simulink model "FullModelAddANN_Final_ANN_revised"  (R2024b)
settings: Solver=ode4  StartTime=0.0  StopTime=40  FixedStep=1e-5  RelTol=1e-3
values from neighbouring files (symbols this model uses):
  Dp = 2.506338228783948e3    (= 2506.33822878)    [FullModelAddANNm_Final.m]    (also in main_opal_ann_control.m)
  Dq = 1.033099625954584    (= 1.03309962595)    [FullModelAddANNm_Final.m]    (also in main_opal_ann_control.m)
  Kp = 0.006383815167581    (= 0.00638381516758)    [FullModelAddANNm_Final.m]    (also in main_opal_ann_control.m)
  Kq = 0.076670166944346    (= 0.0766701669443)    [FullModelAddANNm_Final.m]    (also in main_opal_ann_control.m)
undefined symbols (not defined in the file or in its folder): Filter, Ls, params
libraries: neural x88, spsCurrentMeasurementLib x6, spsParallelRLCBranchLib x6, spsIGBTDiodeLib x6, spsMeanLib x6, spsSeriesRLCBranchLib x6, simulink x4, spsVoltageMeasurementLib x4, spsVariableInductorLib x3, spsVariableResistorLib x3, spsDCVoltageSourceLib x1, spsThreePhaseSourceLib x1
(part 3 of 11)

== system FullModelAddANN_Final_ANN_revised/Feed-Forward Neural Network_strength/Process Input 1 ==
  x : Inport  PortDimensions=200
      mask Display: e = 0.06;c1 = [120 230 180]/255;c2 = ([120 230 180]+0)/(256+128);c3 = ([120 230 180]+128)/(256+128);patch([0 1 1 0],[0 0 1 1],c1);patch([0 1 1 1-e 1-e 0+e],[0 0 1 1-e 0+e 0+e],c2);patch([0 0 1 1-e 0+e 0+e],[0 1 1 1-e 1-e 0+e],c3);plot([0 1 1 0 0],[0 0 1 1 0]);
  mapminmax : neural/Processing Functions/mapminmax  xmin=[-8.56223999999999918486537353601;0.341988000000000014200196574166;11.4306000000000000937916411203;18.8948999999999998067323758733;33.501600000000003376499080332;44.2207999999999969986674841493;53.7240999999999999658939486835;67.3171999999999997044142219238;78.7112999999999942701833788306;88.2877000000000009549694368616;87.0142000000000024328983272426;84.2195999999999997953636921011;75.1424999999999982946974341758;70.2459000000000060026650317013;62.8965999999999993974597600754;58.1272000000000019781509763561;53.039000000000001477928890381;47.5546000000000006480149750132;39.1567999999999969418240652885;34.2475999999999984879650583025;24.8386999999999993349319993285;21.4954000000000000625277607469;15.5536999999999991928234521765;6.39240999999999992553512129234;2.04654999999999986926013662014;-1.18479000000000000980548975349;-8.32602999999999937585926090833;-16.5778999999999996362021192908;-17.0478999999999984993337420747;-28.4237999999999999545252649114;-36.734499999999997044142219238;-41.9243999999999985561771609355;-51.339199999999998169641912682;-60.2991000000000028080648917239;-64.033100000000004570210876409;-68.9287999999999954070517560467;-74.5424000000000006593836587854;-81.1367000000000047066350816749;-86.5153999999999996362021192908;-88.4420999999999963847585604526;-95.1997000000000070940586738288;-95.5378999999999933834260446019;-99.909199999999998453859006986;-101.362999999999999545252649114;-102.371999999999999886313162278;-105.39300000000000068212102633;-108.334999999999993747223925311;-107.676000000000001932676241267;-105.603999999999999204192135949;-106.033000000000001250555214938;-109.465999999999993974597600754;-107.385000000000005115907697473;-110.787000000000006139089236967;-108.763000000000005229594535194;-111.801000000000001932676241267;-116.733999999999994656718627084;-124.862999999999999545252649114;-132.080999999999988858689903282;-139.818999999999988403942552395;-149.477000000000003865352482535;-155.419000000000011141310096718;-162.912000000000006139089236967;-172.710000000000007958078640513;-174.960000000000007958078640513;-176.641999999999995907273842022;-175.318000000000012050804798491;-171.712999999999993860910763033;-175.141999999999995907273842022;-176.205999999999988858689903282;-178.522999999999996134647517465;-178.052999999999997271515894681;-177.605999999999994543031789362;-176.187999999999988176568876952;-177.283999999999991814547684044;-176.68899999999999295141606126;-172.467999999999989313437254168;-171.126000000000004774847184308;-169.0970000000000084128259914;-171.228000000000008640199666843;-171.382000000000005002220859751;-170.621000000000009322320693173;-165.554000000000002046363078989;-158.830000000000012505552149378;-153.207999999999998408384271897;-144.509999999999990905052982271;-137.977000000000003865352482535;-128.074000000000012278178473935;-118.063000000000002387423592154;-109.509000000000000341060513165;-98.0019000000000062300387071446;-86.757999999999995566213328857;-77.2938999999999936107997200452;-68.6098999999999961119101499207;-57.2740999999999971237230056431;-49.8582999999999998408384271897;-41.8474000000000003751665644813;-34.7081999999999979422682372387;-28.5457999999999998408384271897;-22.813300000000001688249540166;-13.833600000000000562749846722;-6.93552000000000035129232855979;-5.91626000000000029643842935911;-4.71670999999999995822008713731;-4.42295000000000015916157281026;-4.29441999999999968196107147378;-3.89672000000000018360424292041;-3.41660999999999992482457855658;-2.41442999999999985405452207488;-1.00232999999999994322763541277;0.7520130000000000425330881626;2.50716999999999989867660588061;4.16727000000000025181634555338;5.89646000000000025664803615655;7.19420999999999999374722392531;7.83779000000000003467448550509;8.51986999999999916610704531195;9.02068000000000047577941586496;9.4842700000000004223466021358;9.89752000000000009549694368616;10.2754999999999991899812812335;10.6089000000000002188471626141;10.906800000000000494537744089 ...(+2559 chars)]  xmax=[111.865999999999999658939486835;112.992000000000004433786671143;112.234999999999999431565811392;109.850999999999999090505298227;113.064999999999997726263245568;118.135999999999995679900166579;124.359999999999999431565811392;132.878999999999990677679306827;140.645000000000010231815394945;148.348000000000013187673175707;156.0970000000000084128259914;164.181000000000011596057447605;170.609000000000008867573342286;175.45699999999999363353708759;177.248999999999995225152815692;173.300000000000011368683772162;172.157000000000010686562745832;173.884999999999990905052982271;176.134999999999990905052982271;177.842000000000012960299500264;176.912000000000006139089236967;178.641999999999995907273842022;178.368999999999999772626324557;179.169000000000011141310096718;175.943999999999988403942552395;173.278999999999996362021192908;172.058999999999997498889570124;169.233000000000004092726157978;171.375;170.43899999999999295141606126;171.050000000000011368683772162;164.754999999999995452526491135;159.145000000000010231815394945;152.873999999999995225152815692;144.052999999999997271515894681;135.844999999999998863131622784;127.575999999999993406163412146;118.522999999999996134647517465;110.171000000000006480149750132;98.8944999999999936335370875895;87.4979000000000013415046851151;78.2850999999999999090505298227;68.0520999999999958163243718445;57.8346999999999979991116560996;49.7299000000000006593836587854;40.7706000000000017280399333686;34.8459999999999965325514494907;29.2646000000000015006662579253;23.2098000000000013187673175707;14.4864999999999994884092302527;7.16436999999999990507149050245;-0.0668678000000000050118131866839;-8.32135000000000069064753915882;-18.791399999999999437250153278;-32.2524999999999977262632455677;-44.6839999999999974988895701244;-56.7535000000000025011104298756;-67.7192000000000007275957614183;-77.1479999999999961346475174651;-89.4813999999999936107997200452;-85.4127000000000009549694368616;-80.3586999999999989086063578725;-74.9572000000000002728484105319;-69.0717999999999960891727823764;-66.0060000000000002273736754432;-55.3436999999999983401721692644;-44.1308000000000006934897101019;-44.1448999999999998067323758733;-34.423099999999998033217707416;-27.5173999999999985277554515051;-18.9917000000000015802470443305;-12.0957000000000007844391802792;-8.20207000000000086004092736403;-4.99021999999999987807086654357;2.17446999999999990293986229517;3.31111000000000021969981389702;10.0512999999999994571453498793;17.7323999999999983856469043531;24.8491999999999997328359313542;36.8487000000000008981260180008;42.3740999999999985448084771633;48.3299000000000020804691303056;57.7278999999999982151166477706;60.8676000000000030354385671671;69.3426000000000044565240386873;74.2934000000000054342308430932;80.8464000000000027057467377745;85.4224999999999994315658113919;87.5735999999999989995558280498;91.5768000000000057525539887138;95.8619999999999947704054648057;99.7070999999999969531927490607;103.042000000000001591615728103;105.320999999999997953636921011;107.885000000000005115907697473;102.995999999999995111465977971;107.939999999999997726263245568;111.680000000000006821210263297;107.954999999999998294697434176;110.293999999999996930455381516;42.4363000000000027966962079518;43.5176000000000016143530956469;44.9217000000000012960299500264;46.1379999999999981241671775933;47.2503999999999990677679306827;48.1154999999999972715158946812;48.8096000000000032059688237496;49.3333999999999974761522025801;49.6741999999999990222931955941;49.8036999999999991928234521765;49.6799000000000035015546018258;49.3725000000000022737367544323;48.8558000000000021145751816221;48.1681999999999987949195201509;47.2317999999999997839950083289;46.0728999999999970782482705545;44.7411000000000029785951483063;43.2085000000000007958078640513;41.4568999999999974193087837193;39.5840000000000031832314562052;37.5833999999999974761522025801;35.4305999999999983174348017201;33.1876000000000033196556614712;32.280999999999998806288203923;32.3111999999999994770405464806 ...(+2416 chars)]  ymin=-1  ymax=1
  p : Outport  PortDimensions=200
      mask Display: e = 0.06;c1 = [120 230 180]/255;c2 = ([120 230 180]+0)/(256+128);c3 = ([120 230 180]+128)/(256+128);patch([0 1 1 0],[0 0 1 1],c1);patch([0 1 1 1-e 1-e 0+e],[0 0 1 1-e 0+e 0+e],c2);patch([0 0 1 1-e 0+e 0+e],[0 1 1 1-e 1-e 0+e],c3);plot([0 1 1 0 0],[0 0 1 1 0]);
  wires:
  x/1 -> mapminmax/1
  mapminmax/1 -> p/1

== system FullModelAddANN_Final_ANN_revised/Feed-Forward Neural Network_strength/Process Output 1 ==
  a : Inport  PortDimensions=2
      mask Display: e = 0.06;c1 = [120 230 180]/255;c2 = ([120 230 180]+0)/(256+128);c3 = ([120 230 180]+128)/(256+128);patch([0 1 1 0],[0 0 1 1],c1);patch([0 1 1 1-e 1-e 0+e],[0 0 1 1-e 0+e 0+e],c2);patch([0 0 1 1-e 0+e 0+e],[0 1 1 1-e 1-e 0+e],c3);plot([0 1 1 0 0],[0 0 1 1 0]);
  mapminmax_reverse : neural/Processing Functions/mapminmax_reverse  xmin=[1.77370000000000005435651928565;0.0371483000000000021523227644593]  xmax=[11.5290999999999996816768543795;0.241464000000000011958434242842]  ymin=-1  ymax=1
  y : Outport  PortDimensions=2
      mask Display: e = 0.06;c1 = [120 230 180]/255;c2 = ([120 230 180]+0)/(256+128);c3 = ([120 230 180]+128)/(256+128);patch([0 1 1 0],[0 0 1 1],c1);patch([0 1 1 1-e 1-e 0+e],[0 0 1 1-e 0+e 0+e],c2);patch([0 0 1 1-e 0+e 0+e],[0 1 1 1-e 1-e 0+e],c3);plot([0 1 1 0 0],[0 0 1 1 0]);
  wires:
  a/1 -> mapminmax_reverse/1
  mapminmax_reverse/1 -> y/1

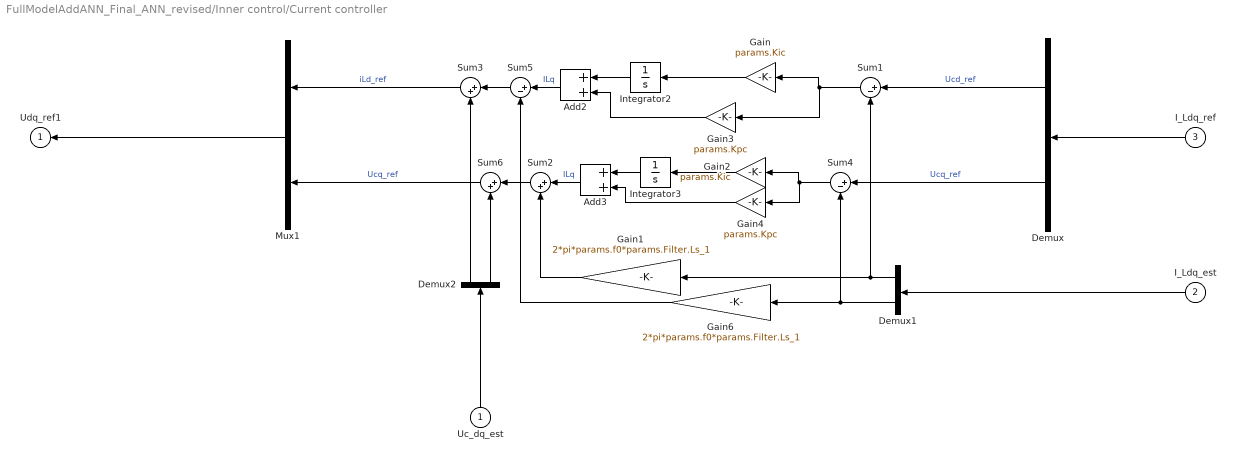
== system FullModelAddANN_Final_ANN_revised/Inner control/Current controller ==
  Uc_dq_est : Inport
  I_Ldq_est : Inport  Port=2
  I_Ldq_ref : Inport  Port=3
  Add2 : Sum
  Add3 : Sum
  Demux : Demux  Outputs=2
  Demux1 : Demux  Outputs=2
  Demux2 : Demux  Outputs=2
  Gain : Gain  Gain=params.Kic
  Gain1 : Gain  Gain=2*pi*params.f0*params.Filter.Ls_1
  Gain2 : Gain  Gain=params.Kic
  Gain3 : Gain  Gain=params.Kpc
  Gain4 : Gain  Gain=params.Kpc
  Gain6 : Gain  Gain=2*pi*params.f0*params.Filter.Ls_1
  Integrator2 : Integrator
  Integrator3 : Integrator
  Mux1 : Mux  Inputs=2
  Sum1 : Sum  Inputs=|+-
  Sum2 : Sum  Inputs=|++
  Sum3 : Sum  Inputs=|++
  Sum4 : Sum  Inputs=|+-
  Sum5 : Sum  Inputs=|+-
  Sum6 : Sum  Inputs=|++
  Udq_ref1 : Outport  InitialOutput=0  VectorParamsAs1DForOutWhenUnconnected=off
  wires:
  I_Ldq_ref/1 -> Demux/1
  Demux2/2 -> Sum6/2
  Sum2/1 -> Sum6/1
  I_Ldq_est/1 -> Demux1/1
  Sum3/1 -> Mux1/1  "iLd_ref"
  Demux/2 -> Sum4/1  "Ucq_ref"
  Gain1/1 -> Sum2/2
  Sum6/1 -> Mux1/2  "Ucq_ref"
  Demux2/1 -> Sum3/2
  Sum5/1 -> Sum3/1
  Mux1/1 -> Udq_ref1/1
  Gain6/1 -> Sum5/2
  Uc_dq_est/1 -> Demux2/1
  Demux1/2 -> Gain6/1, Sum4/2
  Demux/1 -> Sum1/1  "Ucd_ref"
  Demux1/1 -> Sum1/2, Gain1/1
  Add2/1 -> Sum5/1  "ILq"
  Add3/1 -> Sum2/1  "ILq"
  Integrator2/1 -> Add2/1
  Integrator3/1 -> Add3/1
  Gain/1 -> Integrator2/1
  Sum1/1 -> Gain3/1, Gain/1
  Gain2/1 -> Integrator3/1
  Sum4/1 -> Gain4/1, Gain2/1
  Gain3/1 -> Add2/2
  Gain4/1 -> Add3/2

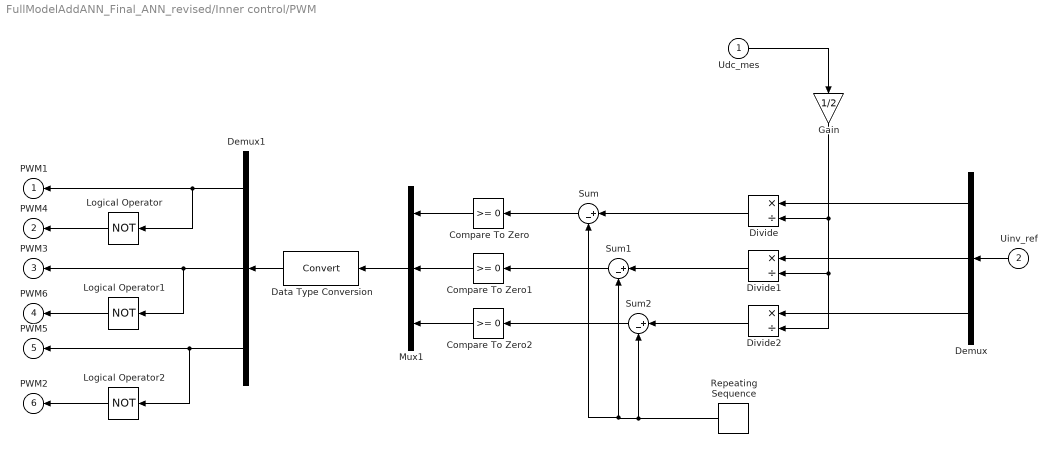
== system FullModelAddANN_Final_ANN_revised/Inner control/PWM ==
  Udc_mes : Inport
  Uinv_ref : Inport  Port=2
  Compare To Zero : simulink/Logic and Bit Operations/Compare To Zero  relop=>=  OutDataTypeStr=boolean
  Compare To Zero1 : simulink/Logic and Bit Operations/Compare To Zero  relop=>=  OutDataTypeStr=boolean
  Compare To Zero2 : simulink/Logic and Bit Operations/Compare To Zero  relop=>=  OutDataTypeStr=boolean
  Data Type Conversion : DataTypeConversion  SaturateOnIntegerOverflow=off  RndMeth=Floor
  Demux : Demux  Outputs=3
  Demux1 : Demux  Outputs=3
  Divide : Product  Inputs=*/
  Divide1 : Product  Inputs=*/
  Divide2 : Product  Inputs=*/
  Gain : Gain  Gain=1/2
  Logical Operator : Logic  Operator=NOT  AllPortsSameDT=off  OutDataTypeStr=boolean
  Logical Operator1 : Logic  Operator=NOT  AllPortsSameDT=off  OutDataTypeStr=boolean
  Logical Operator2 : Logic  Operator=NOT  AllPortsSameDT=off  OutDataTypeStr=boolean
  Mux1 : Mux  Inputs=3
  Repeating Sequence : simulink/Sources/Repeating Sequence  rep_seq_t=[0 params.Ts/2 params.Ts]  rep_seq_y=[-1 1 -1]
  Sum : Sum  Inputs=|+-
  Sum1 : Sum  Inputs=|+-
  Sum2 : Sum  Inputs=|+-
  PWM1 : Outport  InitialOutput=0  VectorParamsAs1DForOutWhenUnconnected=off
  "PWM4 " : Outport  Port=2  InitialOutput=0  VectorParamsAs1DForOutWhenUnconnected=off
  PWM3 : Outport  Port=3  InitialOutput=0  VectorParamsAs1DForOutWhenUnconnected=off
  "PWM6 " : Outport  Port=4  InitialOutput=0  VectorParamsAs1DForOutWhenUnconnected=off
  PWM5 : Outport  Port=5  InitialOutput=0  VectorParamsAs1DForOutWhenUnconnected=off
  PWM2 : Outport  Port=6  InitialOutput=0  VectorParamsAs1DForOutWhenUnconnected=off
  wires:
  Repeating Sequence/1 -> Sum/2, Sum1/2, Sum2/2
  Sum1/1 -> Compare To Zero1/1
  Mux1/1 -> Data Type Conversion/1
  Divide2/1 -> Sum2/1
  Divide/1 -> Sum/1
  Logical Operator/1 -> "PWM4 "/1
  Sum2/1 -> Compare To Zero2/1
  Divide1/1 -> Sum1/1
  Demux/1 -> Divide/1
  Uinv_ref/1 -> Demux/1
  Demux1/2 -> PWM3/1, Logical Operator1/1
  Demux1/3 -> PWM5/1, Logical Operator2/1
  Compare To Zero2/1 -> Mux1/3
  Compare To Zero1/1 -> Mux1/2
  Demux/2 -> Divide1/1
  Logical Operator2/1 -> PWM2/1
  Logical Operator1/1 -> "PWM6 "/1
  Udc_mes/1 -> Gain/1
  Demux/3 -> Divide2/1
  Sum/1 -> Compare To Zero/1
  Gain/1 -> Divide/2, Divide1/2, Divide2/2
  Demux1/1 -> PWM1/1, Logical Operator/1
  Data Type Conversion/1 -> Demux1/1
  Compare To Zero/1 -> Mux1/1

== system FullModelAddANN_Final_ANN_revised/Inner control/Subsystem1 ==
  Uc_abc : Inport
  wt : Inport  Port=2
  Demux : Demux  Outputs=3
  Mux1 : Mux  Inputs=2
  Subsystem1 : Subsystem
  Subsystem2 : Subsystem
  Uc_dq_est : Outport  InitialOutput=0  VectorParamsAs1DForOutWhenUnconnected=off
  wires:
  Mux1/1 -> Uc_dq_est/1
  wt/1 -> Subsystem2/3(wt)
  Demux/3 -> Subsystem1/3(xc)
  Subsystem2/1(xd) -> Mux1/1
  Subsystem1/2(xbeta) -> Subsystem2/2(xbeta)
  Demux/1 -> Subsystem1/1(xa)
  Uc_abc/1 -> Demux/1
  Subsystem1/1(xalpha) -> Subsystem2/1(xalpha)
  Demux/2 -> Subsystem1/2(xb)
  Subsystem2/2(xq) -> Mux1/2

== system FullModelAddANN_Final_ANN_revised/Inner control/Subsystem3 ==
  IL_abc : Inport
  wt : Inport  Port=2
  Demux : Demux  Outputs=3
  Mux1 : Mux  Inputs=2
  Subsystem1 : Subsystem
  Subsystem2 : Subsystem
  IL_dq_est : Outport  InitialOutput=0  VectorParamsAs1DForOutWhenUnconnected=off
  wires:
  Demux/3 -> Subsystem1/3(xc)
  IL_abc/1 -> Demux/1
  wt/1 -> Subsystem2/3(wt)
  Demux/1 -> Subsystem1/1(xa)
  Subsystem1/2(xbeta) -> Subsystem2/2(xbeta)
  Mux1/1 -> IL_dq_est/1
  Demux/2 -> Subsystem1/2(xb)
  Subsystem1/1(xalpha) -> Subsystem2/1(xalpha)
  Subsystem2/2(xq) -> Mux1/2
  Subsystem2/1(xd) -> Mux1/1

== system FullModelAddANN_Final_ANN_revised/Inner control/Subsystem4 ==
  Uc_abc : Inport
  wt : Inport  Port=2
  Demux : Demux  Outputs=3
  Mux1 : Mux  Inputs=2
  Subsystem1 : Subsystem
  Subsystem2 : Subsystem
  Uc_dq_est : Outport  InitialOutput=0  VectorParamsAs1DForOutWhenUnconnected=off
  wires:
  Subsystem2/2(xq) -> Mux1/2
  Demux/2 -> Subsystem1/2(xb)
  Subsystem1/1(xalpha) -> Subsystem2/1(xalpha)
  Uc_abc/1 -> Demux/1
  Demux/1 -> Subsystem1/1(xa)
  Subsystem1/2(xbeta) -> Subsystem2/2(xbeta)
  Subsystem2/1(xd) -> Mux1/1
  Demux/3 -> Subsystem1/3(xc)
  wt/1 -> Subsystem2/3(wt)
  Mux1/1 -> Uc_dq_est/1

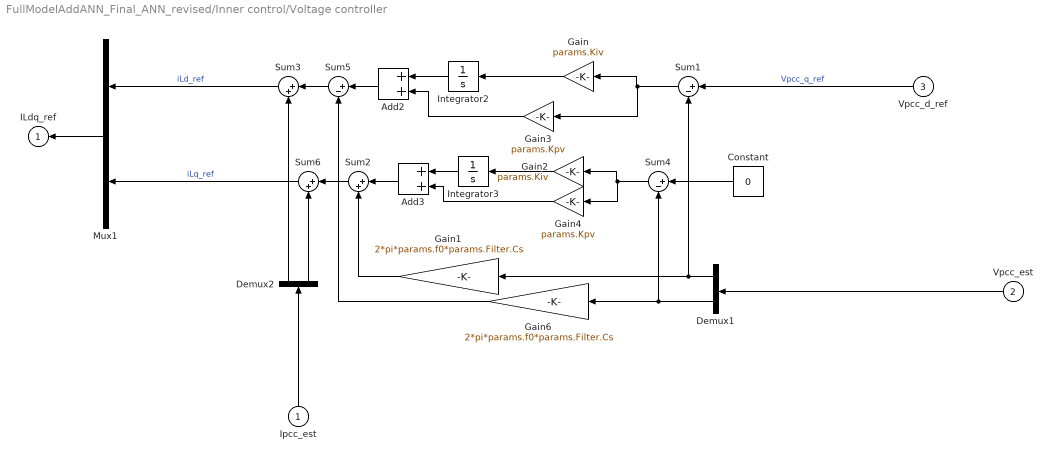
== system FullModelAddANN_Final_ANN_revised/Inner control/Voltage controller ==
  Ipcc_est : Inport
  Vpcc_est : Inport  Port=2
  Vpcc_d_ref : Inport  Port=3
  Add2 : Sum
  Add3 : Sum
  Constant : Constant  Value=0
  Demux1 : Demux  Outputs=2
  Demux2 : Demux  Outputs=2
  Gain : Gain  Gain=params.Kiv
  Gain1 : Gain  Gain=2*pi*params.f0*params.Filter.Cs
  Gain2 : Gain  Gain=params.Kiv
  Gain3 : Gain  Gain=params.Kpv
  Gain4 : Gain  Gain=params.Kpv
  Gain6 : Gain  Gain=2*pi*params.f0*params.Filter.Cs
  Integrator2 : Integrator
  Integrator3 : Integrator
  Mux1 : Mux  Inputs=2
  Sum1 : Sum  Inputs=|+-
  Sum2 : Sum  Inputs=|++
  Sum3 : Sum  Inputs=|++
  Sum4 : Sum  Inputs=|+-
  Sum5 : Sum  Inputs=|+-
  Sum6 : Sum  Inputs=|++
  ILdq_ref : Outport  InitialOutput=0  VectorParamsAs1DForOutWhenUnconnected=off
  wires:
  Gain4/1 -> Add3/2
  Gain3/1 -> Add2/2
  Sum4/1 -> Gain2/1, Gain4/1
  Gain2/1 -> Integrator3/1
  Sum1/1 -> Gain/1, Gain3/1
  Gain/1 -> Integrator2/1
  Integrator3/1 -> Add3/1
  Integrator2/1 -> Add2/1
  Add3/1 -> Sum2/1
  Add2/1 -> Sum5/1
  Demux1/1 -> Gain1/1, Sum1/2
  Demux1/2 -> Sum4/2, Gain6/1
  Ipcc_est/1 -> Demux2/1
  Gain6/1 -> Sum5/2
  Mux1/1 -> ILdq_ref/1
  Sum5/1 -> Sum3/1
  Demux2/1 -> Sum3/2
  Sum6/1 -> Mux1/2  "iLq_ref"
  Gain1/1 -> Sum2/2
  Sum3/1 -> Mux1/1  "iLd_ref"
  Vpcc_est/1 -> Demux1/1
  Sum2/1 -> Sum6/1
  Demux2/2 -> Sum6/2
  Vpcc_d_ref/1 -> Sum1/1  "Vpcc_q_ref"
  Constant/1 -> Sum4/1

== system FullModelAddANN_Final_ANN_revised/Inner control/dq-abc ==
  Udq_ref : Inport
  wt : Inport  Port=2
  Subsystem2 : Subsystem
  Subsystem3 : Subsystem
  Uinv_ref1 : Outport  InitialOutput=0  VectorParamsAs1DForOutWhenUnconnected=off
  wires:
  wt/1 -> Subsystem2/2(wt)
  Subsystem2/1(xalbe) -> Subsystem3/1(xalbe)
  Subsystem3/1(xabc) -> Uinv_ref1/1
  Udq_ref/1 -> Subsystem2/1(xdq)

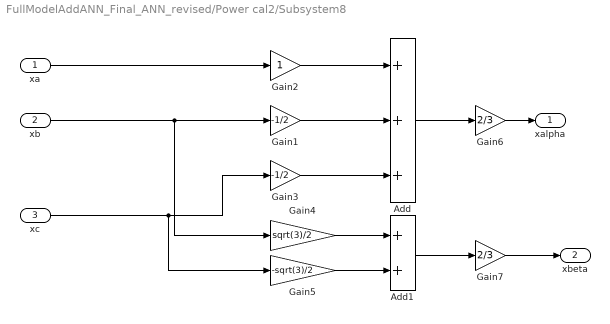
== system FullModelAddANN_Final_ANN_revised/Power cal2/Subsystem8 ==
  xa : Inport
  xb : Inport  Port=2
  xc : Inport  Port=3
  Add : Sum  Inputs=+++
  Add1 : Sum
  Gain1 : Gain  Gain=-1/2
  Gain2 : Gain
  Gain3 : Gain  Gain=-1/2
  Gain4 : Gain  Gain=sqrt(3)/2
  Gain5 : Gain  Gain=-sqrt(3)/2
  Gain6 : Gain  Gain=2/3
  Gain7 : Gain  Gain=2/3
  xalpha : Outport  VectorParamsAs1DForOutWhenUnconnected=off
  xbeta : Outport  Port=2  VectorParamsAs1DForOutWhenUnconnected=off
  wires:
  xc/1 -> Gain5/1, Gain3/1
  Gain6/1 -> xalpha/1
  Add1/1 -> Gain7/1
  Gain3/1 -> Add/3
  Gain1/1 -> Add/2
  xb/1 -> Gain4/1, Gain1/1
  Gain5/1 -> Add1/2
  Gain2/1 -> Add/1
  Add/1 -> Gain6/1
  Gain4/1 -> Add1/1
  Gain7/1 -> xbeta/1
  xa/1 -> Gain2/1

== system FullModelAddANN_Final_ANN_revised/Power cal2/Subsystem9 ==
  xa : Inport
  xb : Inport  Port=2
  xc : Inport  Port=3
  Add : Sum  Inputs=+++
  Add1 : Sum
  Gain1 : Gain  Gain=-1/2
  Gain2 : Gain
  Gain3 : Gain  Gain=-1/2
  Gain4 : Gain  Gain=sqrt(3)/2
  Gain5 : Gain  Gain=-sqrt(3)/2
  Gain6 : Gain  Gain=2/3
  Gain7 : Gain  Gain=2/3
  xalpha : Outport  VectorParamsAs1DForOutWhenUnconnected=off
  xbeta : Outport  Port=2  VectorParamsAs1DForOutWhenUnconnected=off
  wires:
  xa/1 -> Gain2/1
  Gain7/1 -> xbeta/1
  Gain4/1 -> Add1/1
  Add/1 -> Gain6/1
  Gain2/1 -> Add/1
  Gain5/1 -> Add1/2
  xb/1 -> Gain1/1, Gain4/1
  Gain1/1 -> Add/2
  Gain3/1 -> Add/3
  Add1/1 -> Gain7/1
  Gain6/1 -> xalpha/1
  xc/1 -> Gain3/1, Gain5/1

== system FullModelAddANN_Final_ANN_revised/Power cal2/p3 ==
  Alpha : Inport
  Beta : Inport  Port=2
  xalpha : Inport  Port=3
  xbeta : Inport  Port=4
  Add : Sum
  Gain : Gain  Gain=3/2
  Product : Product
  Product1 : Product
  deltay1 : Outport
  wires:
  Product1/1 -> Add/2
  Gain/1 -> deltay1/1
  Product/1 -> Add/1
  Add/1 -> Gain/1
  Alpha/1 -> Product/1
  xalpha/1 -> Product/2
  Beta/1 -> Product1/1
  xbeta/1 -> Product1/2

== system FullModelAddANN_Final_ANN_revised/Power cal2/q3 ==
  Alpha : Inport
  Beta : Inport  Port=2
  xalpha : Inport  Port=3
  xbeta : Inport  Port=4
  Add : Sum  Inputs=+-
  Gain : Gain  Gain=3/2
  Product : Product
  Product1 : Product
  deltay2 : Outport
  wires:
  Add/1 -> Gain/1
  Product/1 -> Add/1
  Gain/1 -> deltay2/1
  Product1/1 -> Add/2
  Beta/1 -> Product/1
  xalpha/1 -> Product/2
  Alpha/1 -> Product1/1
  xbeta/1 -> Product1/2

== system FullModelAddANN_Final_ANN_revised/Power_control/Subsystem6 ==
  deltay1 : Inport
  deltay2 : Inport  Port=2
  In1 : Inport  Port=3
  In3 : Inport  Port=4
  In2 : Inport  Port=5
  Demux10 : Demux  Outputs=2
  K : Gain  Gain=[-17.7280896028731 21.0955836516851 -166.273972820736 -21.116209501605 -8436.7525192577;-266.263993446395 3.66786652155975 256.175641614485 -97.6658040979501 3301.94041224969]  Multiplication=Matrix(K*u)
  Mux7 : Mux  Inputs=5
  Out1 : Outport
  Out2 : Outport  Port=2
  wires:
  In2/1 -> Mux7/5
  In3/1 -> Mux7/4
  Demux10/2 -> Out2/1
  deltay1/1 -> Mux7/1
  deltay2/1 -> Mux7/2
  In1/1 -> Mux7/3
  Demux10/1 -> Out1/1
  K/1 -> Demux10/1
  Mux7/1 -> K/1

== system FullModelAddANN_Final_ANN_revised/Feed-Forward Neural Network2/Layer 1/Delays 1 ==
  "p{1}" : Inport  PortDimensions=200
      mask Display: e = 0.06;c1 = [120 230 180]/255;c2 = ([120 230 180]+0)/(256+128);c3 = ([120 230 180]+128)/(256+128);patch([0 1 1 0],[0 0 1 1],c1);patch([0 1 1 1-e 1-e 0+e],[0 0 1 1-e 0+e 0+e],c2);patch([0 0 1 1-e 0+e 0+e],[0 1 1 1-e 1-e 0+e],c3);plot([0 1 1 0 0],[0 0 1 1 0]);
  mux : Mux  Inputs=1
      mask Display: e = 0.06;c1 = [120 150 230]/255;c2 = ([120 150 230]+0)/383;c3 = ([120 150 230]+128)/383;patch([0 1 1 0],[0 0 1 1],c1);patch([0 1 1 1-e 1-e 0+e],[0 0 1 1-e 0+e 0+e],c2);patch([0 0 1 1-e 0+e 0+e],[0 1 1 1-e 1-e 0+e],c3);plot([0 1 1 0 0],[0 0 1 1 0]);disp('Mux')
  "pd{1,1}" : Outport
      mask Display: e = 0.06;c1 = [120 230 180]/255;c2 = ([120 230 180]+0)/(256+128);c3 = ([120 230 180]+128)/(256+128);patch([0 1 1 0],[0 0 1 1],c1);patch([0 1 1 1-e 1-e 0+e],[0 0 1 1-e 0+e 0+e],c2);patch([0 0 1 1-e 0+e 0+e],[0 1 1 1-e 1-e 0+e],c3);plot([0 1 1 0 0],[0 0 1 1 0]);
  wires:
  "p{1}"/1 -> mux/1
  mux/1 -> "pd{1,1}"/1
